simulink model "Blocks_for_copy_R2023a"  (R2023a)
settings: Solver=VariableStepAuto  StartTime=0.0  StopTime=10.0  RelTol=1e-3
values from neighbouring files (symbols this model uses):
  IMU_w_b_bias = IMU_var_bias_matrix(:,2)    [EKF.m]
  P0 = diag([P0_ph_meas,P0_th_meas,P0_ps_meas,P0_bias_wp,P0_bias_wq,P0_bias_wr])    [EKF.m]
  Q = diag([q_phi,q_theta,q_psi, q_bias_w_b,q_bias_w_b,q_bias_w_b])    [EKF.m]
  q_bias_w_b = 1e-2    (= 0.01)    [EKF.m]
  R = diag([r_th_meas,r_th_meas,r_ps_meas])    [EKF.m]
  Rbody_frd = [cos(angleZ) -sin(angleZ)   0 ... (first row only)    [EKF.m]
  Rbody_ned = Rbody_frd*Rfrd_ned    [EKF.m]
  Ts_EKF_integr = 0.01    [EKF.m]
  Ts_EKF_meas = 0.01    [EKF.m]
  Ts_slk = 0.01    [main_matteo.m]    (also in quadcopterMain.m)
  x0EKF = [ph0;th0;ps0;bias_wp0;bias_wq0;bias_wr0]    [EKF.m]
undefined symbols (not defined in the file or in its folder): acc_pole, RPY_pole
settings Model: Creator=teoma  LastModifiedBy=teoma

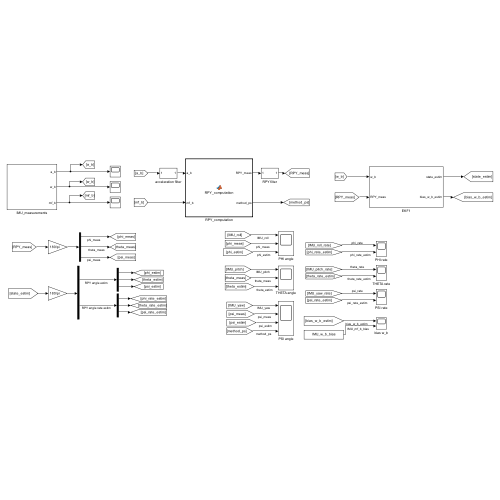
[thumbnail: Simulink's stored preview of the top-level diagram]
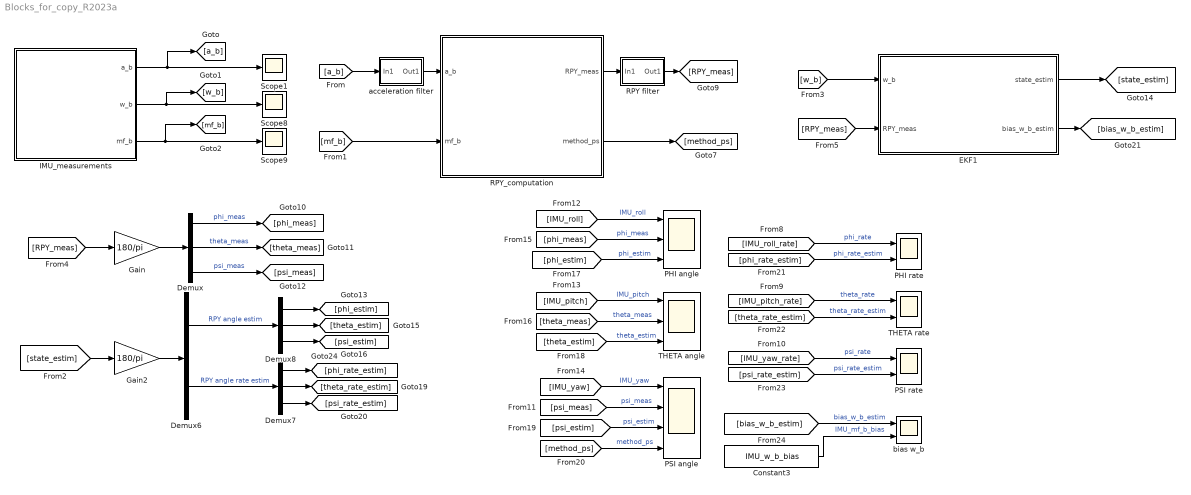
== system Blocks_for_copy_R2023a ==
  Constant3 : Constant  Value=IMU_w_b_bias
  Demux : Demux  Outputs=3
  Demux6 : Demux  Outputs=2
  Demux7 : Demux  Outputs=3
  Demux8 : Demux  Outputs=3
  EKF1 : Subsystem
  Gain : Gain  Gain=180/pi
  Gain2 : Gain  Gain=180/pi
  IMU_measurements : Subsystem
  PHI angle : Scope  NumInputPorts=3
  PHI rate : Scope  NumInputPorts=2
  PSI angle : Scope  NumInputPorts=4
  PSI rate : Scope  NumInputPorts=2
  RPY filter : Subsystem  mask{p=RPY_pole}
      mask prompts: p "pole (p)"
  RPY_computation : MATLAB Function  TreatAsAtomicUnit=on
  Scope1 : Scope
  Scope8 : Scope
  Scope9 : Scope
  THETA angle : Scope  NumInputPorts=3
  THETA rate : Scope  NumInputPorts=2
  acceleration filter : Subsystem  mask{p=acc_pole}
      mask prompts: p "pole (p)"
  bias w_b : Scope  NumInputPorts=2
  wires:
  IMU_measurements/2(w_b) -> Scope8/1, [w_b]
  IMU_measurements/1(a_b) -> [a_b], Scope1/1
  IMU_measurements/3(mf_b) -> [mf_b], Scope9/1
  Demux8/2 -> [theta_estim]
  Demux/2 -> [theta_meas]  "theta_meas"
  Gain2/1 -> Demux6/1
  Demux6/2 -> Demux7/1  "RPY angle rate estim"
  Demux7/2 -> [theta_rate_estim]
  [RPY_meas] -> EKF1/2(RPY_meas)
  [IMU_pitch_rate] -> THETA rate/1  "theta_rate"
  Gain/1 -> Demux/1
  [phi_estim] -> PHI angle/3  "phi_estim"
  [theta_estim] -> THETA angle/3  "theta_estim"
  RPY_computation/1(RPY_meas) -> RPY filter/1(In1)
  Demux8/3 -> [psi_estim]
  Demux7/3 -> [psi_rate_estim]
  Demux7/1 -> [phi_rate_estim]
  Demux/3 -> [psi_meas]  "psi_meas"
  [state_estim] -> Gain2/1
  [IMU_roll] -> PHI angle/1  "IMU_roll"
  [theta_meas] -> THETA angle/2  "theta_meas"
  Demux6/1 -> Demux8/1  "RPY angle estim"
  [phi_rate_estim] -> PHI rate/2  "phi_rate_estim"
  [phi_meas] -> PHI angle/2  "phi_meas"
  [method_ps] -> PSI angle/4  "method_ps"
  RPY_computation/2(method_ps) -> [method_ps]
  [IMU_roll_rate] -> PHI rate/1  "phi_rate"
  acceleration filter/1(Out1) -> RPY_computation/1(a_b)
  [mf_b] -> RPY_computation/2(mf_b)
  [psi_estim] -> PSI angle/3  "psi_estim"
  [a_b] -> acceleration filter/1(In1)
  [IMU_yaw] -> PSI angle/1  "IMU_yaw"
  [psi_meas] -> PSI angle/2  "psi_meas"
  [psi_rate_estim] -> PSI rate/2  "psi_rate_estim"
  [theta_rate_estim] -> THETA rate/2  "theta_rate_estim"
  [w_b] -> EKF1/1(w_b)
  RPY filter/1(Out1) -> [RPY_meas]
  [IMU_pitch] -> THETA angle/1  "IMU_pitch"
  EKF1/2(bias_w_b_estim) -> [bias_w_b_estim]
  [IMU_yaw_rate] -> PSI rate/1  "psi_rate"
  Demux8/1 -> [phi_estim]
  Constant3/1 -> bias w_b/2  "IMU_mf_b_bias"
  EKF1/1(state_estim) -> [state_estim]
  Demux/1 -> [phi_meas]  "phi_meas"
  [bias_w_b_estim] -> bias w_b/1  "bias_w_b_estim"
  [RPY_meas] -> Gain/1

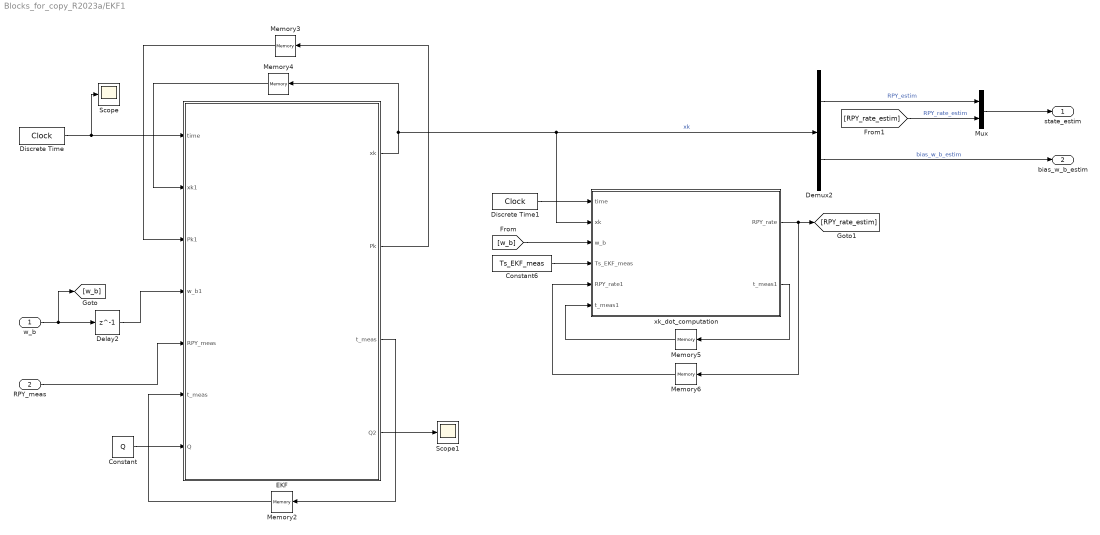
== system Blocks_for_copy_R2023a/EKF1 ==
  w_b : Inport
  RPY_meas : Inport  Port=2
  Constant : Constant  Value=Q
  Constant6 : Constant  Value=Ts_EKF_meas
  Delay2 : Delay  DelayLength=1  SampleTime=Ts_EKF_meas
  Demux2 : Demux  Outputs=2
  Discrete Time : DigitalClock  SampleTime=Ts_slk
  Discrete Time1 : DigitalClock  SampleTime=Ts_slk
  EKF : MATLAB Function  TreatAsAtomicUnit=on
  Memory2 : Memory
  Memory3 : Memory  InitialCondition=P0
  Memory4 : Memory  InitialCondition=x0EKF
  Memory5 : Memory
  Memory6 : Memory
  Mux : Mux  Inputs=2
  Scope : Scope
  Scope1 : Scope
  xk_dot_computation : MATLAB Function  TreatAsAtomicUnit=on
  state_estim : Outport
  bias_w_b_estim : Outport  Port=2
  wires:
  w_b/1 -> Delay2/1, [w_b]
  EKF/2(Pk) -> Memory3/1
  Memory2/1 -> EKF/6("t_meas ")
  EKF/3(t_meas) -> Memory2/1
  RPY_meas/1 -> EKF/5(RPY_meas)
  Discrete Time/1 -> Scope/1, EKF/1(time)
  Memory3/1 -> EKF/3(Pk1)
  Delay2/1 -> EKF/4(w_b1)
  Memory4/1 -> EKF/2(xk1)
  xk_dot_computation/2(t_meas1) -> Memory5/1
  Memory5/1 -> xk_dot_computation/6("t_meas1 ")
  Memory6/1 -> xk_dot_computation/5(RPY_rate1)
  xk_dot_computation/1(RPY_rate) -> [RPY_rate_estim], Memory6/1
  [w_b] -> xk_dot_computation/3(w_b)
  Discrete Time1/1 -> xk_dot_computation/1(time)
  Demux2/2 -> bias_w_b_estim/1  "bias_w_b_estim"
  Demux2/1 -> Mux/1  "RPY_estim"
  EKF/1(xk) -> xk_dot_computation/2(xk), Demux2/1, Memory4/1  "xk"
  [RPY_rate_estim] -> Mux/2  "RPY_rate_estim"
  Mux/1 -> state_estim/1
  Constant6/1 -> xk_dot_computation/4(Ts_EKF_meas)
  EKF/4(Q2) -> Scope1/1
  Constant/1 -> EKF/7(Q)

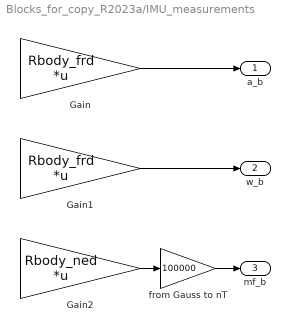
== system Blocks_for_copy_R2023a/IMU_measurements ==
  Gain : Gain  Gain=Rbody_frd  Multiplication=Matrix(K*u) (u vector)
  Gain1 : Gain  Gain=Rbody_frd  Multiplication=Matrix(K*u) (u vector)
  Gain2 : Gain  Gain=Rbody_ned  Multiplication=Matrix(K*u) (u vector)
  from Gauss to nT : Gain  Gain=100000
  a_b : Outport
  w_b : Outport  Port=2
  mf_b : Outport  Port=3
  wires:
  Gain/1 -> a_b/1
  Gain1/1 -> w_b/1
  from Gauss to nT/1 -> mf_b/1
  Gain2/1 -> from Gauss to nT/1
  ? -> Gain2/1

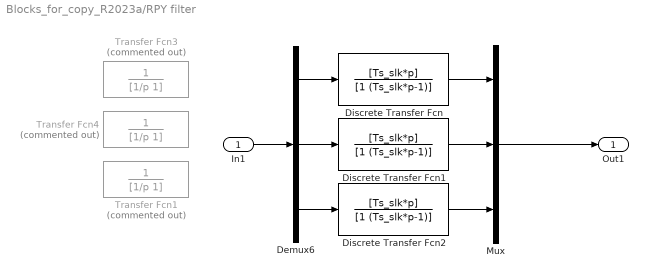
== system Blocks_for_copy_R2023a/RPY filter ==
  In1 : Inport
  Demux6 : Demux  Outputs=3
  Discrete Transfer Fcn : DiscreteTransferFcn  Numerator=[Ts_slk*p]  Denominator=[1 (Ts_slk*p-1)]
  Discrete Transfer Fcn1 : DiscreteTransferFcn  Numerator=[Ts_slk*p]  Denominator=[1 (Ts_slk*p-1)]
  Discrete Transfer Fcn2 : DiscreteTransferFcn  Numerator=[Ts_slk*p]  Denominator=[1 (Ts_slk*p-1)]
  Mux : Mux  Inputs=3
  Transfer Fcn1 : TransferFcn  Commented=on  Denominator=[1/p 1]
  Transfer Fcn3 : TransferFcn  Commented=on  Denominator=[1/p 1]
  Transfer Fcn4 : TransferFcn  Commented=on  Denominator=[1/p 1]
  Out1 : Outport
  wires:
  Discrete Transfer Fcn/1 -> Mux/1
  Discrete Transfer Fcn2/1 -> Mux/3
  Demux6/3 -> Discrete Transfer Fcn2/1
  Demux6/1 -> Discrete Transfer Fcn/1
  Demux6/2 -> Discrete Transfer Fcn1/1
  In1/1 -> Demux6/1
  Mux/1 -> Out1/1
  Discrete Transfer Fcn1/1 -> Mux/2

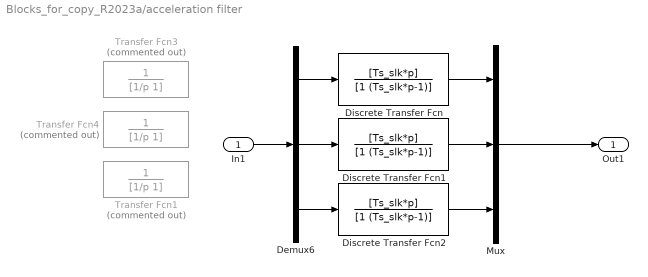
== system Blocks_for_copy_R2023a/acceleration filter ==
  In1 : Inport
  Demux6 : Demux  Outputs=3
  Discrete Transfer Fcn : DiscreteTransferFcn  Numerator=[Ts_slk*p]  Denominator=[1 (Ts_slk*p-1)]
  Discrete Transfer Fcn1 : DiscreteTransferFcn  Numerator=[Ts_slk*p]  Denominator=[1 (Ts_slk*p-1)]
  Discrete Transfer Fcn2 : DiscreteTransferFcn  Numerator=[Ts_slk*p]  Denominator=[1 (Ts_slk*p-1)]
  Mux : Mux  Inputs=3
  Transfer Fcn1 : TransferFcn  Commented=on  Denominator=[1/p 1]
  Transfer Fcn3 : TransferFcn  Commented=on  Denominator=[1/p 1]
  Transfer Fcn4 : TransferFcn  Commented=on  Denominator=[1/p 1]
  Out1 : Outport
  wires:
  Discrete Transfer Fcn1/1 -> Mux/2
  Demux6/3 -> Discrete Transfer Fcn2/1
  Mux/1 -> Out1/1
  Discrete Transfer Fcn2/1 -> Mux/3
  Discrete Transfer Fcn/1 -> Mux/1
  In1/1 -> Demux6/1
  Demux6/1 -> Discrete Transfer Fcn/1
  Demux6/2 -> Discrete Transfer Fcn1/1

== matlab function Blocks_for_copy_R2023a/EKF1/EKF ==
  data: time input; xk1 input; Pk1 input; w_b1 input; RPY_meas input; t_meas input; xk output; Pk output; t_meas output; R parameter; Q input; Ts_EKF_integr parameter; Ts_EKF_meas parameter; q_bias_w_b parameter; Q2 output
function [xk,Pk,t_meas,Q2] = EKF(time,xk1,Pk1,w_b1,RPY_meas,t_meas,R, Q, Ts_EKF_integr, Ts_EKF_meas, q_bias_w_b)

% if time <= 0.01
%     xk = ;
%     Pk = ;
%     t_meas = 0;

% if Q(4,4) == q_bias_w_b && max(abs([xk1(4,1),xk1(5,1),xk1(6,1)])) < 0.1 
% if time < 2
%     Q = Q1;
% else 
%     Q = Q1;
%     Q(4,4) = Q(4,4)*1e-20;
%     Q(5,5) = Q(5,5)*1e-20;
%     Q(6,6) = Q(6,6)*1e-20;
% end

if time - t_meas >= Ts_EKF_meas
    t_meas = time;

  % INTEGRATION STEP
    % initial condition
    xt1         =       xk1;                        % initial condition for the state
    Pt1         =       Pk1;                        % initial condition for matrix P
    wp1         =       w_b1(1,1);                  % past value of the p-dir of angular velocity w
    wq1         =       w_b1(2,1);                  % past value of the q-dir of angular velocity w
    wr1         =       w_b1(3,1);                  % past value of the r-dir of angular velocity w
    % integration loop
    Nstep       = floor(Ts_EKF_meas/Ts_EKF_integr); % number of integration steps to performe in the t_meas time windows
    xt          = zeros(6,1);
    Pt          = zeros(6,6);
    for i = 1:1:Nstep
        % state extraction
            phi         =       xt1(1,1);           % roll angle (rad)
            theta       =       xt1(2,1);           % pitch angle (rad)
            psi         =       xt1(3,1);           % yaw angle (rad)  
            bias_wp     =       xt1(4,1);           % bias of p-dir of angular velocity w
            bias_wq     =       xt1(5,1);           % bias of q-dir of angular velocity w
            bias_wr     =       xt1(6,1);           % bias of r-dir of angular velocity w
        
            cph         =       cos(phi);
            cth         =       cos(theta);
            cps         =       cos(psi);
            sph         =       sin(phi);
            sth         =       sin(theta);
            sps         =       sin(psi);
            tth         =       sth/cth;
        % integration
            Mf = [1,    sph*tth,    cph*tth,    0,  0,  0;
                  0,    cph,        -sph,       0,  0,  0;
                  0,    sph/cth,    cph/cth,    0,  0,  0;
                  0,    0,          0,          0,  0,  0;
                  0,    0,          0,          0,  0,  0;
                  0,    0,          0,          0,  0,  0;];
            Z1 = [wp1-bias_wp; wq1-bias_wq; wr1-bias_wr; bias_wp; bias_wq; bias_wr;];
            f = Mf*Z1;
            xt = xt1 + Ts_EKF_integr*f;
        
            A1 = [cph*tth*(wq1-bias_wq)-sph*tth*(wr1-bias_wr),(sph*(wq1-bias_wq)+cph*(wr1-bias_wr))/cth^2,  0,  -1, -sph*tth,   -cph*tth;];
            A2 = [-sph*(wq1-bias_wq)-cph*(wr1-bias_wr),   0,  0,  0,  -cph,   sph;];
            A3 = [cph*(wq1-bias_wq)/cth-sph*(wr1-bias_wr)/cth, (sth/cth^2)*(sph*(wq1-bias_wq)+cph*(wr1-bias_wr)),   0,  0,  -sph/cth,   -cph/cth;];
            A4 = [0,    0,  0,  0,  0,  0;];
            A5 = [0,    0,  0,  0,  0,  0;];
            A6 = [0,    0,  0,  0,  0,  0;];
            At1 = [A1; A2; A3; A4; A5; A6;];
            Pt = Pt1 + Ts_EKF_integr*(At1*Pt1 + Pt1*At1' + Q);
        % house keeping
            xt1 = xt;
            Pt1 = Pt;
    end
  % MEASUREMENT STEP
    Ck = [eye(3),zeros(3,3)];
    Lk = Pt*Ck'/(Ck*Pt*Ck' + R);
    xk = xt + Lk*(RPY_meas - Ck*xt);
    Pk = (eye(6) - Lk*Ck)*Pt;
else
    xk = xk1;
    Pk = Pk1;
end

Q2 = diag(Q);
end

== matlab function Blocks_for_copy_R2023a/EKF1/xk_dot_computation ==
  data: time input; xk input; w_b input; Ts_EKF_meas input; RPY_rate1 input; RPY_rate output; t_meas1 input; t_meas1 output
function [RPY_rate,t_meas1] = xk_dot_computation(time,xk,w_b,Ts_EKF_meas,RPY_rate1,t_meas1)
RPY_rate = zeros(3,1);
if time == 0
    t_meas1 = 0;
end
if time - t_meas1 >= Ts_EKF_meas || time == 0
    wp          =       w_b(1,1);        % p-dir of angular velocity w
    wq          =       w_b(2,1);        % q-dir of angular velocity w
    wr          =       w_b(3,1);        % r-dir of angular velocity w

    phi         =       xk(1,1);         %  roll angle (rad)
    theta       =       xk(2,1);         %  pitch angle (rad)
    psi         =       xk(3,1);         %  yaw angle (rad)  
    bias_wp     =       xk(4,1)*0;         % bias of p-dir of angular velocity w
    bias_wq     =       xk(5,1)*0;         % bias of q-dir of angular velocity w
    bias_wr     =       xk(6,1)*0;         % bias of r-dir of angular velocity w

    cph         =       cos(phi);
    cth         =       cos(theta);
    cps         =       cos(psi);
    sph         =       sin(phi);
    sth         =       sin(theta);
    sps         =       sin(psi);
    tth         =       sth/cth;

    % integration step
    t_meas1 = time;
    W_eta = [1,    sph*tth,    cph*tth;
             0,    cph,        -sph;
             0,    sph/cth,    cph/cth;];
    w_b_corrected = [wp-bias_wp; wq-bias_wq; wr-bias_wr;];
    RPY_rate = W_eta*w_b_corrected;
else
    RPY_rate = RPY_rate1;
end
end

== matlab function Blocks_for_copy_R2023a/RPY_computation ==
  data: a_b input; mf_b input; RPY_meas output; method_ps output
function [RPY_meas,method_ps]   = RPY_computation(a_b,mf_b)
% description:
% - a_b             = measured linear acceleration in body-frame
% - w_b             = measured angular velocity in body-frame
% - mf_b            = measured magnetic field in body-frame
% - mf              = measured magnetic field in body-inertia
% - a_b_disturbe    = linear velocity measurement-noise
% - w_b_disturbe    = angular velocity measurement-noise
% - mf_b_disturbe   = magnetic field measurement-noise

% -------------------------------------------------------------------------------------------
% observation: the following computation works only if the angles
% phi,theta,psy are withing angles (-pi/2,+pi/2) (this is an open set, pi/2 is excluded)
% -------------------------------------------------------------------------------------------

a_b = -1*a_b;       % need to adjust the sign to use atan2() function correctly

% phi computation
ph_meas = atan2(a_b(2), a_b(3));
sph = sin(ph_meas);
cph = cos(ph_meas);

% theta computation
th_meas = atan2(-a_b(1), (a_b(2)*sph + a_b(3)*cph));
sth = sin(th_meas);
cth = cos(th_meas);

% psi computation
% if abs(sin(th_meas)) > 0.15  % sin(th) != 0 
%     method_ps = 1;
%     ps_meas_numerator   = (sth*cph*mf_b(2) - sth*sph*mf_b(3))/(-sth);       % don't modify
%     ps_meas_denominator = (-sph*mf_b(2) - cph*mf_b(3) + cth*mf_u)/(-sth);   % don't modify
%     ps_meas = atan2(ps_meas_numerator, ps_meas_denominator);
% else                        % sin(th) == 0
%     method_ps = 2;
%     ps_meas_numerator   = (mf_b(2) - cth*sph*mf_u)*(-cth);
%     ps_meas_denominator = cph*mf_b(1);
%     ps_meas = atan2(ps_meas_numerator, ps_meas_denominator);
% end

ps_meas_num   = mf_b(3)*sph - mf_b(2)*cph;
ps_meas_den = mf_b(1)*cth + mf_b(2)*sth*sph + mf_b(3)*sth*cph;
ps_meas = atan2(ps_meas_num, ps_meas_den);
method_ps = 1;
% if abs(ps_meas_den) > 0.01
%     ps_meas = atan2(ps_meas_num, ps_meas_den);
%     method_ps = 1;
% else
%     if ps_meas_num > 0 
%         ps_meas = pi/2;
%     else
%         ps_meas = -pi/2;
%     end
%     method_ps = 2;
% end

RPY_meas = [ph_meas;th_meas;ps_meas];
